simulink model "ArduCopter_MinnieLindiCopterFtc"  (R2018b)
settings: Solver=FixedStepDiscrete  StartTime=0.0  StopTime=1000  FixedStep=lindi.ts  RelTol=1e-4
libraries: ardupilot_custom_controller_lib x2, copterFtc_lib x2, simulink x2, lindiCopter_lib x1, axes_transformation_lib x1
settings Model: DataTypeOverride=Single  DataTypeOverrideAppliesTo=Floating-point  Creator=Yannic  LastModifiedBy=yannic
settings SolverCC: ZeroCrossControl=DisableAll
settings DataIOCC: LimitDataPoints=on  SaveOutput=off  SaveTime=off  ReturnWorkspaceOutputs=on
settings OptimizationCC: DefaultParameterBehavior=Inlined  UseFloatMulNetSlope=on  DefaultUnderspecifiedDataType=single  InlineInvariantSignals=on  PassReuseOutputArgsAs=Individual arguments  ZeroExternalMemoryAtStartup=off  ZeroInternalMemoryAtStartup=off  NoFixptDivByZeroProtection=on  EfficientFloat2IntCast=on  LifeSpan=1  OptimizeBlockOrder=speed  DifferentSizesBufferReuse=on
settings DebuggingCC: ReadBeforeWriteMsg=DisableAll  WriteAfterWriteMsg=DisableAll  WriteAfterReadMsg=DisableAll  MultiTaskDSMMsg=none  ParameterTunabilityLossMsg=error  AllowSymbolicDim=off  LibraryContextMissingDiagnostic=none  SFUnexpectedBacktrackingDiag=warning  SFNoUnconditionalDefaultTransitionDiag=warning  SFExecutionAtInitializationDiag=none
settings HardwareCC: ProdBitPerPointer=32  ProdBitPerSizeT=32  ProdBitPerPtrDiffT=32  ProdLargestAtomicInteger=Long  ProdWordSize=32  ProdHWDeviceType=ARM Compatible->ARM 7
settings ModelReferenceCC: UpdateModelReferenceTargets=IfOutOfDate  PropagateSignalLabelsOutOfModel=off
settings SFSimCC: SFSimEcho=off  SimUseLocalCustomCode=off  MATLABDynamicMemAlloc=off
settings RTWCC: SystemTargetFile=ert.tlc  GenCodeOnly=on  TemplateMakefile=ert_default_tmf  GenerateReport=on  RTWUseLocalCustomCode=off  IncludeHyperlinkInReport=on  LaunchReport=on  TargetLang=C++  GenerateTraceInfo=on  GenerateTraceReport=on  GenerateTraceReportSl=on  GenerateTraceReportSf=on  GenerateTraceReportEml=on
settings CodeAppCC: ForceParamTrailComments=on  IgnoreCustomStorageClasses=off  OperatorAnnotations=on  SimulinkDataObjDesc=on  SFDataObjDesc=on  CustomSymbolStrGlobalVar=rt$N$M  CustomSymbolStrType=$N$M  CustomSymbolStrFcn=$N$M$F  CustomSymbolStrMacro=$N$M  InsertBlockDesc=on
settings ERTTargetCC: TargetLangStandard=C++03 (ISO)  GenerateSampleERTMain=on  IncludeMdlTerminateFcn=off  CombineSignalStateStructs=on  SuppressErrorStatus=on  SupportAbsoluteTime=off  MultiInstanceERTCode=on  CodeInterfacePackaging=C++ class  SupportNonFinite=off  SupportComplex=off  SupportVariableSizeSignals=on  ERTHeaderFileRootName=MatlabController$E  ERTSourceFileRootName=MatlabController$E  ERTDataFileRootName=MatlabController_data  InlinedParameterPlacement=NonHierarchical  RootIOFormat=Structure reference  ERTCustomFileTemplate=example_file_process.tlc  ERTFilePackagingFormat=CompactWithDataFile
settings ConfigComp: CovMetricSettings=dw  CovHtmlReporting=on  CovSaveCumulativeToWorkspaceVar=on  CovSaveSingleToWorkspaceVar=on  CovExternalEMLEnable=off

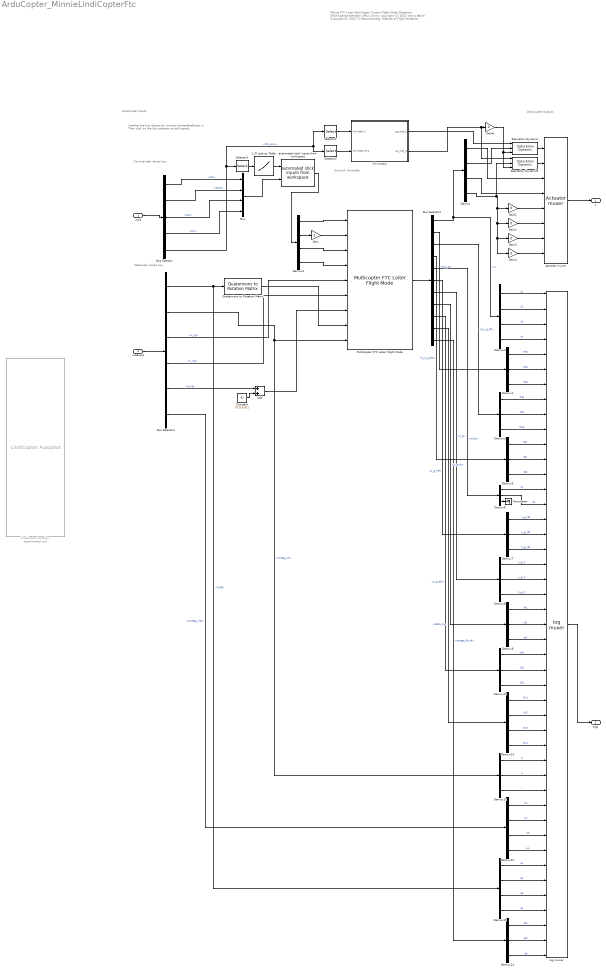
== system ArduCopter_MinnieLindiCopterFtc ==
  note: Measured values bus
  note: Initialize the bus objects by running initInterfaceBuses.m.
      | Then click on the bus selectors to add signals.
  note: Commanded values bus
  note: ArduCopter Inputs
  note: ArduCopter Outputs
  note: Simulink Controller
  note: Minnie FTC Loiter ArduCopter Custom Flight Mode
      |
      | Disclamer:
      | SPDX-License-Identifier: GPL-2.0-only
      |
      | Copyright (C) 2022 Yannic Beyer
      | Copyright (C) 2022 TU Braunschweig, Institute of Flight Guidance
  cmd : Inport  OutDataTypeStr=Bus: cmdBus
  measure : Inport  Port=2  OutDataTypeStr=Bus: measureBus
  1-D Lookup Table : Lookup_n-D  NumberOfTableDimensions=1  BreakpointsForDimension1=[1000;2000]  Table=[0;1]  InternalRulePriority=Speed  RndMeth=Simplest  InputSameDT=on
  Actuator muxer : ardupilot_custom_controller_lib/Actuator muxer
      settings: SourceProductName=LADAC
  Add : Sum
  Bus Selector : BusSelector  OutputSignals=roll,pitch,yaw,thr,RC_pwm
  Bus Selector1 : BusSelector  OutputSignals=q_bg,omega_Kb,s_Kg,V_Kg,a_Kg,omega_mot
  Bus Selector2 : BusSelector  OutputSignals=inner_loop_indi.u,pos_cntrl.error.e_s_g,pos_cntrl.error.e_s_g_dt,pos_cntrl.error.e_s_g_dt2,atti_cntrl.reference.reduced_attitude.n_flip,pos_cntrl.reference.s_g_ref,pos_cntrl.measure.s_g,pos_cntrl.measure.s_g_dt,pos_cntrl.measure.s_g_dt2,inner_loop_indi.Delta_nu,atti_cntrl.measure.omega_Kb_dt
  Constant : Constant  Value=[0;0;9.81]
  Demux{,2,4,12..13,15} (6 alike) : Demux
  Demux{1,3,5..11,14} (10 alike) : Demux  Outputs=3
  Gain : Gain  Gain=-1
  Gain{1..4,6} (5 alike) : Gain  Gain=0
  LindiCopter Autopilot : lindiCopter_lib/LindiCopter Autopilot  Commented=on  ap=lindi
      settings: SourceProductName=LADAC
  Multicopter FTC Loiter Flight Mode : copterFtc_lib/Multicopter FTC Loiter Flight Mode  fm=lindi
  Mux : Mux
  Quaternions to Rotation Matrix : axes_transformation_lib/Quaternions to Rotation Matrix  SystemSampleTime=-1
      settings: SourceProductName=LADAC
  Saturation Dynamic : simulink/Discontinuities/Saturation Dynamic  OutMin=[]  OutMax=[]  OutDataTypeStr=Inherit: Same as second input  OutDataType=fixdt(1, 16)  OutScaling=2^-10  DoSatur=off
  Saturation Dynamic1 : simulink/Discontinuities/Saturation Dynamic  OutMin=[]  OutMax=[]  OutDataTypeStr=Inherit: Same as second input  OutDataType=fixdt(1, 16)  OutScaling=2^-10  DoSatur=off
  Selector1 : Selector  InputPortWidth=16  IndexOptions=Index vector (dialog)  Indices=7  OutputSizes=1
  Selector2 : Selector  InputPortWidth=16  IndexOptions=Index vector (dialog)  Indices=8  OutputSizes=1
  Selector3 : Selector  InputPortWidth=16  IndexOptions=Index vector (dialog)  Indices=9  OutputSizes=1
  Terminator : Terminator
  automated stick inputs from workspace : copterFtc_lib/automated stick inputs from workspace  simin=simin
  kill motors : Subsystem
  log muxer : ardupilot_custom_controller_lib/log muxer  batch_name_1='ML1'  num_signals_1=14  batch_name_2='ML2'  num_signals_2=13  batch_name_3='ML3'  num_signals_3=11  batch_name_4='ML4'  num_signals_4=7  batch_name_5='ML5'  num_signals_5=0
      settings: SourceProductName=LADAC
  u : Outport
  logs : Outport  Port=2
  wires:
  cmd/1 -> Bus Selector/1
  measure/1 -> Bus Selector1/1
  Bus Selector/1 -> Mux/1  "<roll>"
  Bus Selector/2 -> Mux/2  "<pitch>"
  Bus Selector/3 -> Mux/3  "<yaw>"
  Bus Selector/4 -> Mux/4  "<thr>"
  Actuator muxer/1 -> u/1
  log muxer/1 -> logs/1
  Demux6/2 -> log muxer/15  "h2"
  Bus Selector/5 -> Selector1/1, Selector2/1, Selector3/1  "<RC_pwm>"
  Demux/4 -> Saturation Dynamic1/2, Gain1/1, Gain4/1, Gain3/1, Gain2/1
  Multicopter FTC Loiter Flight Mode/1 -> Bus Selector2/1
  Demux3/2 -> log muxer/9  "evg"
  Demux1/1 -> log muxer/5  "exg"
  kill motors/1(up_mot_2) -> Saturation Dynamic/1
  Gain1/1 -> Actuator muxer/5
  Gain4/1 -> Actuator muxer/8
  Demux1/3 -> log muxer/7  "ezg"
  Demux1/2 -> log muxer/6  "eyg"
  Gain3/1 -> Actuator muxer/7
  Demux2/2 -> log muxer/2  "u2"
  Bus Selector2/1 -> Demux2/1, Demux/1  "<u>"
  Demux/2 -> Saturation Dynamic/2
  kill motors/2(up_mot_4) -> Saturation Dynamic1/1, Gain6/1
  Demux2/3 -> log muxer/3  "u3"
  Demux3/1 -> log muxer/8  "eug"
  Gain2/1 -> Actuator muxer/6
  Demux/1 -> Actuator muxer/3
  Gain6/1 -> Saturation Dynamic/3, Saturation Dynamic1/3
  Demux2/4 -> log muxer/4  "u4"
  Demux2/1 -> log muxer/1  "u1"
  Saturation Dynamic/1 -> Actuator muxer/1
  Saturation Dynamic1/1 -> Actuator muxer/2
  Demux/3 -> Actuator muxer/4
  Demux3/3 -> log muxer/10  "ewg"
  Demux5/2 -> log muxer/12  "eay"
  Demux5/3 -> log muxer/13  "eaz"
  Demux6/1 -> log muxer/14  "h1"
  Bus Selector1/1 -> Quaternions to Rotation Matrix/1, Demux15/1  "<q_bg>"
  Quaternions to Rotation Matrix/1 -> Multicopter FTC Loiter Flight Mode/8
  Gain/1 -> Multicopter FTC Loiter Flight Mode/2
  Demux4/4 -> Multicopter FTC Loiter Flight Mode/4
  Bus Selector2/2 -> Demux1/1  "<e_s_g>"
  Bus Selector2/3 -> Demux3/1  "<e_s_g_dt>"
  Selector3/1 -> 1-D Lookup Table/1
  1-D Lookup Table/1 -> automated stick inputs from workspace/1
  Mux/1 -> automated stick inputs from workspace/2
  Demux4/2 -> Gain/1
  Demux4/3 -> Multicopter FTC Loiter Flight Mode/3
  Demux4/1 -> Multicopter FTC Loiter Flight Mode/1
  automated stick inputs from workspace/1 -> Demux4/1
  Bus Selector1/5 -> Add/1  "<a_Kg>"
  Bus Selector2/4 -> Demux5/1  "<e_s_g_dt2>"
  Add/1 -> Multicopter FTC Loiter Flight Mode/7
  Constant/1 -> Add/2
  Demux5/1 -> log muxer/11  "eax"
  Bus Selector2/5 -> Demux6/1  "<n_flip>"
  Demux6/3 -> Terminator/1
  Bus Selector2/6 -> Demux7/1  "<s_g_ref>"
  Demux7/1 -> log muxer/16  "x_g_ref"
  Demux7/2 -> log muxer/17  "y_g_ref"
  Demux7/3 -> log muxer/18  "z_g_ref"
  Demux8/1 -> log muxer/19  "x_g_m"
  Demux8/2 -> log muxer/20  "y_g_m"
  Demux8/3 -> log muxer/21  "z_g_m"
  Bus Selector2/7 -> Demux8/1  "<s_g>"
  Bus Selector2/8 -> Demux9/1  "<s_g_dt>"
  Demux9/1 -> log muxer/22  "xd1"
  Demux9/2 -> log muxer/23  "yd1"
  Demux9/3 -> log muxer/24  "zd1"
  Demux10/1 -> log muxer/25  "xd2"
  Demux10/2 -> log muxer/26  "yd2"
  Demux10/3 -> log muxer/27  "zd2"
  Bus Selector2/9 -> Demux10/1  "<s_g_dt2>"
  Demux11/3 -> log muxer/34  "r"
  Demux11/2 -> log muxer/33  "q"
  Demux11/1 -> log muxer/32  "p"
  Demux12/4 -> log muxer/38  "w4"
  Demux12/3 -> log muxer/37  "w3"
  Demux12/2 -> log muxer/36  "w2"
  Demux12/1 -> log muxer/35  "w1"
  Bus Selector1/6 -> Demux12/1  "<omega_mot>"
  Bus Selector2/10 -> Demux13/1  "<Delta_nu>"
  Demux13/1 -> log muxer/28  "Dv1"
  Demux13/2 -> log muxer/29  "Dv2"
  Demux13/3 -> log muxer/30  "Dv3"
  Demux13/4 -> log muxer/31  "Dv4"
  Demux15/1 -> log muxer/39  "q1"
  Demux15/2 -> log muxer/40  "q2"
  Demux15/3 -> log muxer/41  "q3"
  Demux15/4 -> log muxer/42  "q4"
  Demux14/1 -> log muxer/43  "pdt"
  Demux14/2 -> log muxer/44  "qdt"
  Demux14/3 -> log muxer/45  "rdt"
  Bus Selector2/11 -> Demux14/1  "<omega_Kb_dt>"
  Bus Selector1/2 -> Demux11/1, Multicopter FTC Loiter Flight Mode/9  "<omega_Kb>"
  Bus Selector1/3 -> Multicopter FTC Loiter Flight Mode/5  "<s_Kg>"
  Bus Selector1/4 -> Multicopter FTC Loiter Flight Mode/6  "<V_Kg>"
  Selector1/1 -> kill motors/1(kill motor 2)
  Selector2/1 -> kill motors/2(kill motor 2+4)

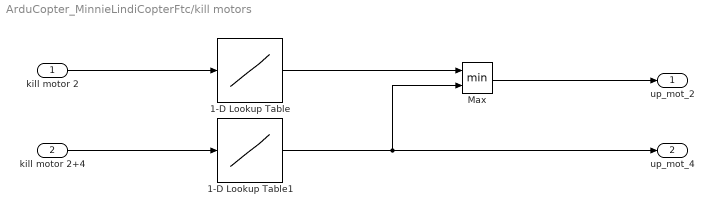
== system ArduCopter_MinnieLindiCopterFtc/kill motors ==
  kill motor 2 : Inport
  kill motor 2+4 : Inport  Port=2
  1-D Lookup Table : Lookup_n-D  NumberOfTableDimensions=1  BreakpointsForDimension1=[1000;2000]  Table=[1;0]  InternalRulePriority=Speed  RndMeth=Simplest  InputSameDT=on
  1-D Lookup Table1 : Lookup_n-D  NumberOfTableDimensions=1  BreakpointsForDimension1=[1000;2000]  Table=[1;0]  InternalRulePriority=Speed  RndMeth=Simplest  InputSameDT=on
  Max : MinMax  Inputs=2
  up_mot_2 : Outport
  up_mot_4 : Outport  Port=2
  wires:
  1-D Lookup Table1/1 -> Max/2, up_mot_4/1
  kill motor 2/1 -> 1-D Lookup Table/1
  kill motor 2+4/1 -> 1-D Lookup Table1/1
  1-D Lookup Table/1 -> Max/1
  Max/1 -> up_mot_2/1
